simulink model "FlightSim"  (Simulink 7.9)
settings: Solver=ode45  StartTime=0.0  StopTime=10.0  RelTol=1e-3
undefined symbols (not defined in the file or in its folder): datcom_out, deg, ft, m, Newton, nfs, rad, Raphson, s, sigbuilder_block
libraries: aerolibconvert2 x12, aerolibadyn x2, aerolibasang x2, aerolibutil x1, simulink x1
(part 2 of 2)

== system FlightSim/6DoF Nonlinear Flight Equations of Motion (Rigid Body)/AngularAcceleration(Omegadot)/Cross Product/Subsystem3 ==
  A : Inport
  B : Inport  Port=2
  Demux : Demux  Outputs=3
  Demux1 : Demux  Outputs=3
  Mux : Mux  Inputs=3
  i x k : Product  SaturateOnIntegerOverflow=on  InputSameDT=on  OutDataTypeStr=Inherit: Same as first input
  j x i : Product  SaturateOnIntegerOverflow=on  InputSameDT=on  OutDataTypeStr=Inherit: Same as first input
  k x j : Product  SaturateOnIntegerOverflow=on  InputSameDT=on  OutDataTypeStr=Inherit: Same as first input
  Out2 : Outport
  wires:
  j x i/1 -> Mux/3
  i x k/1 -> Mux/2
  k x j/1 -> Mux/1
  Mux/1 -> Out2/1
  Demux1/1 -> j x i/2
  Demux/2 -> j x i/1
  Demux1/3 -> i x k/2
  Demux/1 -> i x k/1
  Demux1/2 -> k x j/2
  Demux/3 -> k x j/1
  B/1 -> Demux1/1
  A/1 -> Demux/1

== system FlightSim/6DoF Nonlinear Flight Equations of Motion (Rigid Body)/Linear Acceleration(Vdot)/Cross Product/Subsystem2 ==
  A : Inport
  B : Inport  Port=2
  Demux : Demux  Outputs=3
  Demux1 : Demux  Outputs=3
  Mux : Mux  Inputs=3
  i x j : Product  SaturateOnIntegerOverflow=on  InputSameDT=on  OutDataTypeStr=Inherit: Same as first input
  j x k : Product  SaturateOnIntegerOverflow=on  InputSameDT=on  OutDataTypeStr=Inherit: Same as first input
  k x i : Product  SaturateOnIntegerOverflow=on  InputSameDT=on  OutDataTypeStr=Inherit: Same as first input
  Out1 : Outport
  wires:
  Demux1/3 -> j x k/2
  Demux/2 -> j x k/1
  Demux/3 -> k x i/1
  Demux1/1 -> k x i/2
  Demux1/2 -> i x j/2
  Demux/1 -> i x j/1
  i x j/1 -> Mux/3
  k x i/1 -> Mux/2
  j x k/1 -> Mux/1
  B/1 -> Demux1/1
  A/1 -> Demux/1
  Mux/1 -> Out1/1

== system FlightSim/6DoF Nonlinear Flight Equations of Motion (Rigid Body)/Linear Acceleration(Vdot)/Cross Product/Subsystem3 ==
  A : Inport
  B : Inport  Port=2
  Demux : Demux  Outputs=3
  Demux1 : Demux  Outputs=3
  Mux : Mux  Inputs=3
  i x k : Product  SaturateOnIntegerOverflow=on  InputSameDT=on  OutDataTypeStr=Inherit: Same as first input
  j x i : Product  SaturateOnIntegerOverflow=on  InputSameDT=on  OutDataTypeStr=Inherit: Same as first input
  k x j : Product  SaturateOnIntegerOverflow=on  InputSameDT=on  OutDataTypeStr=Inherit: Same as first input
  Out2 : Outport
  wires:
  j x i/1 -> Mux/3
  i x k/1 -> Mux/2
  k x j/1 -> Mux/1
  Mux/1 -> Out2/1
  Demux1/1 -> j x i/2
  Demux/2 -> j x i/1
  Demux1/3 -> i x k/2
  Demux/1 -> i x k/1
  Demux1/2 -> k x j/2
  Demux/3 -> k x j/1
  B/1 -> Demux1/1
  A/1 -> Demux/1

== system FlightSim/Forces & Moments/Aerodynamic Forces and Moments/Aero Attributes/Dynamic Pressure Calc ==
  Air Density : Inport  PortDimensions=1
  Linear Velocity (Body) : Inport  Port=2  PortDimensions=[3 1]
  0.5*rh : Product  SaturateOnIntegerOverflow=on  InputSameDT=on  OutDataTypeStr=Inherit: Same as first input
  Dot Product : DotProduct  InputSameDT=on  OutDataTypeStr=Inherit: Inherit via internal rule
  Gain : Gain  Gain=0.5  SaturateOnIntegerOverflow=on  OutDataTypeStr=Inherit: Same as input  ParamDataTypeStr=Inherit: Same as input
  V^2 : Abs
  Dynamic Pressure : Outport
  wires:
  Dot Product/1 -> V^2/1
  Linear Velocity (Body)/1 -> Dot Product/2, Dot Product/1
  Air Density/1 -> Gain/1
  V^2/1 -> 0.5*rh/1
  Gain/1 -> 0.5*rh/2
  0.5*rh/1 -> Dynamic Pressure/1

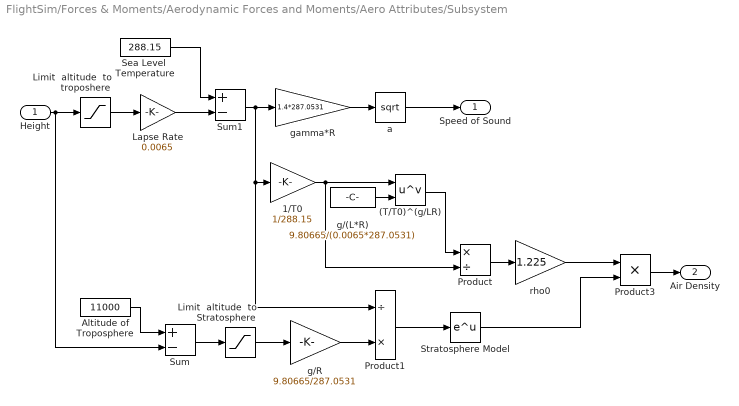
== system FlightSim/Forces & Moments/Aerodynamic Forces and Moments/Aero Attributes/Subsystem ==
  Height : Inport
  "(T/T0)^(g/LR) " : Math  Operator=pow  SaturateOnIntegerOverflow=on
  1/T0 : Gain  Gain=1/288.15  SaturateOnIntegerOverflow=on  OutDataTypeStr=Inherit: Same as input  ParamDataTypeStr=Inherit: Same as input
  Altitude of Troposphere : Constant  Value=11000  OutDataTypeStr=Inherit: Inherit via back propagation
  Lapse Rate : Gain  Gain=0.0065  SaturateOnIntegerOverflow=on  OutDataTypeStr=Inherit: Same as input  ParamDataTypeStr=Inherit: Same as input
  Limit  altitude  to Stratosphere : Saturate  UpperLimit=0  LowerLimit=11000-20000
  Limit  altitude  to troposhere : Saturate  UpperLimit=11000  LowerLimit=0
  Product : Product  Inputs=*/  SaturateOnIntegerOverflow=on  InputSameDT=on  OutDataTypeStr=Inherit: Same as first input
  Product1 : Product  Inputs=/*  SaturateOnIntegerOverflow=on  InputSameDT=on  OutDataTypeStr=Inherit: Same as first input
  Product3 : Product  SaturateOnIntegerOverflow=on  InputSameDT=on  OutDataTypeStr=Inherit: Same as first input
  Sea Level  Temperature : Constant  Value=288.15  OutDataTypeStr=Inherit: Inherit via back propagation
  Stratosphere Model : Math  SaturateOnIntegerOverflow=on
  Sum : Sum  Inputs=+-  SaturateOnIntegerOverflow=on  InputSameDT=on  OutDataTypeStr=Inherit: Same as first input
  Sum1 : Sum  Inputs=+-  SaturateOnIntegerOverflow=on  InputSameDT=on  OutDataTypeStr=Inherit: Same as first input
  a : Sqrt  AlgorithmType=Newton-Raphson  SaturateOnIntegerOverflow=on
  g/(L*R) : Constant  Value=9.80665/(0.0065*287.0531)  OutDataTypeStr=Inherit: Inherit via back propagation
  g/R : Gain  Gain=9.80665/287.0531  SaturateOnIntegerOverflow=on  OutDataTypeStr=Inherit: Same as input  ParamDataTypeStr=Inherit: Same as input
  gamma*R : Gain  Gain=1.4*287.0531  SaturateOnIntegerOverflow=on  OutDataTypeStr=Inherit: Same as input  ParamDataTypeStr=Inherit: Same as input
  rho0 : Gain  Gain=1.225  SaturateOnIntegerOverflow=on  OutDataTypeStr=Inherit: Same as input  ParamDataTypeStr=Inherit: Same as input
  Speed of Sound : Outport  PortDimensions=1
  Air Density : Outport  Port=2  PortDimensions=1
  wires:
  g/(L*R)/1 -> "(T/T0)^(g/LR) "/2
  Height/1 -> Limit  altitude  to troposhere/1, Sum/2
  Limit  altitude  to troposhere/1 -> Lapse Rate/1
  Product/1 -> rho0/1
  "(T/T0)^(g/LR) "/1 -> Product/1
  1/T0/1 -> "(T/T0)^(g/LR) "/1, Product/2
  gamma*R/1 -> a/1
  a/1 -> Speed of Sound/1
  Sum1/1 -> gamma*R/1, 1/T0/1, Product1/1
  Lapse Rate/1 -> Sum1/2
  Sea Level  Temperature/1 -> Sum1/1
  rho0/1 -> Product3/1
  Product3/1 -> Air Density/1
  Stratosphere Model/1 -> Product3/2
  g/R/1 -> Product1/2
  Product1/1 -> Stratosphere Model/1
  Altitude of Troposphere/1 -> Sum/1
  Sum/1 -> Limit  altitude  to Stratosphere/1
  Limit  altitude  to Stratosphere/1 -> g/R/1

== system FlightSim/Forces & Moments/Aerodynamic Forces and Moments/Aero Attributes/Velocity Magnitude ==
  Velocity : Inport
  Dot Product : DotProduct  InputSameDT=on  OutDataTypeStr=Inherit: Inherit via internal rule
  Sqrt : Sqrt  SaturateOnIntegerOverflow=on
  Velocity Magnitude : Outport
  wires:
  Sqrt/1 -> Velocity Magnitude/1  "abs(V)"
  Velocity/1 -> Dot Product/2, Dot Product/1
  Dot Product/1 -> Sqrt/1

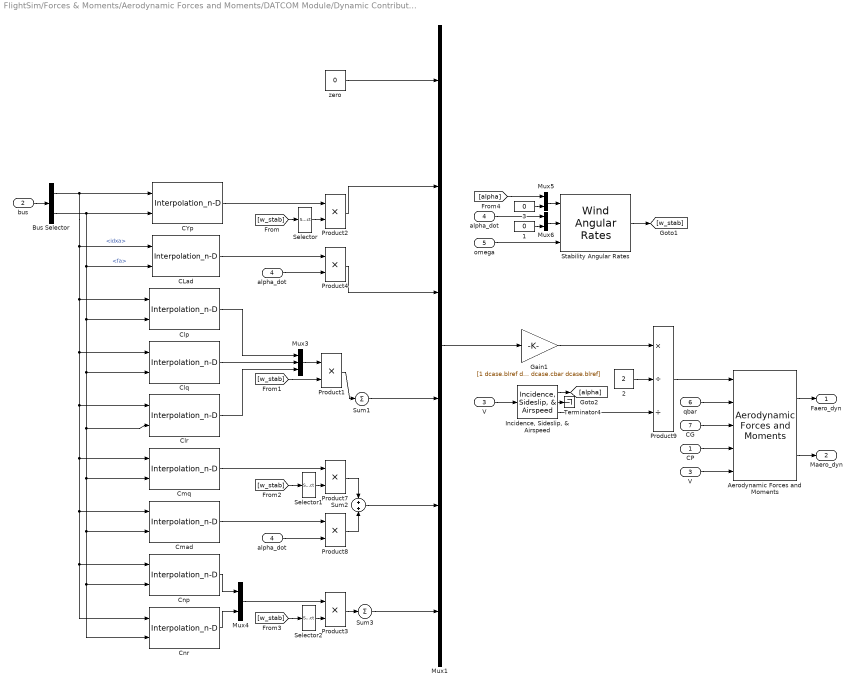
== system FlightSim/Forces & Moments/Aerodynamic Forces and Moments/DATCOM Module/Dynamic Contribution ==
  CP : Inport
  bus : Inport  Port=2
  V : Inport  Port=3
  alpha_dot : Inport  Port=4
  omega : Inport  Port=5
  qbar : Inport  Port=6
  CG : Inport  Port=7
  " V " : InportShadow  Port=3
  " alpha_dot " : InportShadow  Port=4
  1 : Constant  Value=0
  2 : Constant  Value=2
  3 : Constant  Value=0
  Aerodynamic Forces and Moments : aerolibadyn/Aerodynamic Forces and Moments   inputAxes=Stability  outputForceAxes=Body  outputMomentAxes=Body  S=dcase.sref  b=dcase.blref  cbar=dcase.cbar
  Bus Selector : BusSelector  OutputSignals=idxa,fa
  CLad : Interpolation_n-D  NumberOfTableDimensions=1  Table="permute(dcase.clad,[1  2])"  OutDataTypeStr=double
      settings: InputPortMap=u0,u1
  CYp : Interpolation_n-D  NumberOfTableDimensions=1  Table="permute(dcase.cyp,[1  2])"  OutDataTypeStr=double
      settings: InputPortMap=u0,u1
  Clp : Interpolation_n-D  NumberOfTableDimensions=1  Table="permute(dcase.clp,[1  2])"  OutDataTypeStr=double
      settings: InputPortMap=u0,u1
  Clq : Interpolation_n-D  NumberOfTableDimensions=1  Table="permute(dcase.clq,[1  2])"  OutDataTypeStr=double
      settings: InputPortMap=u0,u1
  Clr : Interpolation_n-D  NumberOfTableDimensions=1  Table="permute(dcase.clr,[1  2])"  OutDataTypeStr=double
      settings: InputPortMap=u0,u1
  Cmad : Interpolation_n-D  NumberOfTableDimensions=1  Table="permute(dcase.cmad,[1  2])"  OutDataTypeStr=double
      settings: InputPortMap=u0,u1
  Cmq : Interpolation_n-D  NumberOfTableDimensions=1  Table="permute(dcase.cmq,[1  2])"  OutDataTypeStr=double
      settings: InputPortMap=u0,u1
  Cnp : Interpolation_n-D  NumberOfTableDimensions=1  Table="permute(dcase.cnp,[1  2])"  OutDataTypeStr=double
      settings: InputPortMap=u0,u1
  Cnr : Interpolation_n-D  NumberOfTableDimensions=1  Table="permute(dcase.cnr,[1  2])"  OutDataTypeStr=double
      settings: InputPortMap=u0,u1
  Gain1 : Gain  Gain=[1 dcase.blref dcase.cbar dcase.blref dcase.cbar dcase.blref]
  "Incidence, Sideslip, & Airspeed" : aerolibasang/Incidence, Sideslip, & Airspeed
  Mux1 : Mux  Inputs=6
  Mux3 : Mux  Inputs=3
  Mux4 : Mux  Inputs=2
  Mux5 : Mux  Inputs=2
  Mux6 : Mux  Inputs=2
  Product{1..4,7..8} (6 alike) : Product  RndMeth=Zero
  Product9 : Product  Inputs=*//  RndMeth=Zero
  Selector : Selector  InputPortWidth=3  IndexOptions=Index vector (dialog)  Indices=1  OutputSizes=1
  Selector1 : Selector  InputPortWidth=3  IndexOptions=Index vector (dialog)  Indices=2  OutputSizes=1
  Selector2 : Selector  InputPortWidth=3  IndexOptions=Index vector (dialog)  Indices=[1 3]  OutputSizes=1
  Stability Angular Rates : aerolibasang/Wind Angular Rates
  Sum1 : Sum  Inputs=+
  Sum2 : Sum  Inputs=+|+
  Sum3 : Sum  Inputs=+
  Terminator4 : Terminator
  "alpha_dot " : InportShadow  Port=4
  zero : Constant  Value=0
  Faero_dyn : Outport
  Maero_dyn : Outport  Port=2
  wires:
  bus/1 -> Bus Selector/1
  Mux1/1 -> Gain1/1
  CLad/1 -> Product4/1
  Cnp/1 -> Mux4/1
  Cmq/1 -> Product7/1
  Sum1/1 -> Mux1/4
  Clq/1 -> Mux3/2
  Selector/1 -> Product2/2
  CYp/1 -> Product2/1
  "alpha_dot "/1 -> Product4/2
  [w_stab] -> Selector/1
  Clr/1 -> Mux3/3
  Clp/1 -> Mux3/1
  Mux3/1 -> Product1/1
  [w_stab] -> Product1/2
  Product1/1 -> Sum1/1
  [w_stab] -> Selector1/1
  Selector1/1 -> Product7/2
  Product7/1 -> Sum2/1
  Cmad/1 -> Product8/1
  Product8/1 -> Sum2/2
  alpha_dot/1 -> Product8/2
  Cnr/1 -> Mux4/2
  [w_stab] -> Selector2/1
  Mux4/1 -> Product3/1
  Selector2/1 -> Product3/2
  Sum3/1 -> Mux1/6
  Product3/1 -> Sum3/1
  Gain1/1 -> Product9/1
  Product9/1 -> Aerodynamic Forces and Moments/1
  2/1 -> Product9/2
  V/1 -> "Incidence, Sideslip, & Airspeed"/1
  omega/1 -> Stability Angular Rates/3
  Sum2/1 -> Mux1/5
  Product4/1 -> Mux1/3
  zero/1 -> Mux1/1
  "Incidence, Sideslip, & Airspeed"/3 -> Product9/3
  "Incidence, Sideslip, & Airspeed"/2 -> Terminator4/1
  "Incidence, Sideslip, & Airspeed"/1 -> [alpha]
  Aerodynamic Forces and Moments/1 -> Faero_dyn/1
  qbar/1 -> Aerodynamic Forces and Moments/2
  Aerodynamic Forces and Moments/2 -> Maero_dyn/1
  " V "/1 -> Aerodynamic Forces and Moments/5
  Stability Angular Rates/1 -> [w_stab]
  [alpha] -> Mux5/1
  Mux5/1 -> Stability Angular Rates/1
  Mux6/1 -> Stability Angular Rates/2
  " alpha_dot "/1 -> Mux6/1
  1/1 -> Mux6/2
  CG/1 -> Aerodynamic Forces and Moments/3
  CP/1 -> Aerodynamic Forces and Moments/4
  Bus Selector/1 -> CYp/1, CLad/1, Cnr/1, Cnp/1, Cmad/1, Cmq/1, Clr/1, Clq/1, Clp/1  "<idxa>"
  Bus Selector/2 -> CYp/2, CLad/2, Cnr/2, Cnp/2, Cmad/2, Cmq/2, Clr/2, Clq/2, Clp/2  "<fa>"
  3/1 -> Mux5/2
  Product2/1 -> Mux1/2

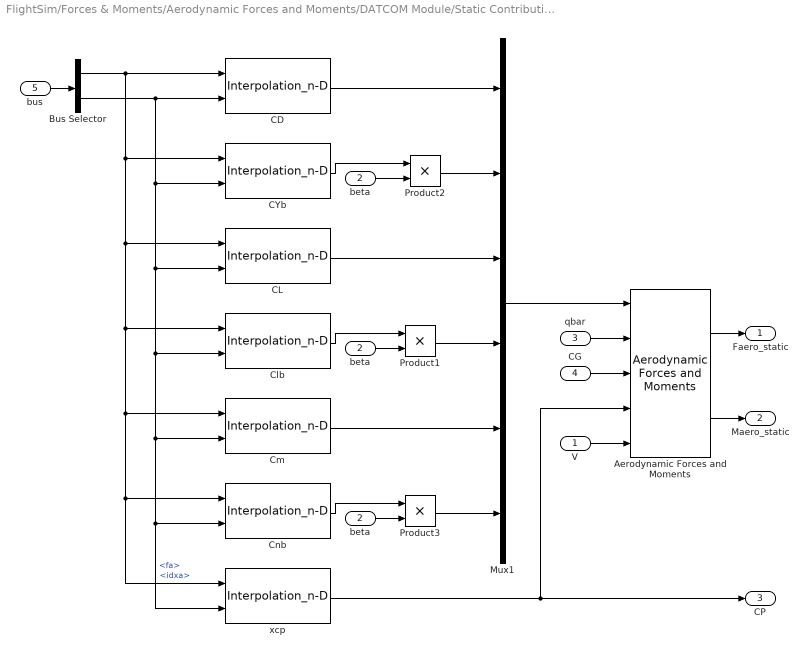
== system FlightSim/Forces & Moments/Aerodynamic Forces and Moments/DATCOM Module/Static Contribution ==
  "V " : Inport
  beta : Inport  Port=2
  qbar : Inport  Port=3
  CG : Inport  Port=4
  bus : Inport  Port=5
  " beta " : InportShadow  Port=2
  Aerodynamic Forces and Moments : aerolibadyn/Aerodynamic Forces and Moments   inputAxes=Stability  outputForceAxes=Body  outputMomentAxes=Body  S=dcase.sref  b=dcase.blref  cbar=dcase.cbar
  Bus Selector : BusSelector  OutputSignals=idxa,fa
  CD : Interpolation_n-D  NumberOfTableDimensions=1  Table=dcase.cd  OutDataTypeStr=double
      settings: InputPortMap=u0,u1
  CL : Interpolation_n-D  NumberOfTableDimensions=1  Table=dcase.cl  OutDataTypeStr=double
      settings: InputPortMap=u0,u1
  CYb : Interpolation_n-D  NumberOfTableDimensions=1  Table=dcase.cyb  OutDataTypeStr=double
      settings: InputPortMap=u0,u1
  Clb : Interpolation_n-D  NumberOfTableDimensions=1  Table=dcase.clb  OutDataTypeStr=double
      settings: InputPortMap=u0,u1
  Cm : Interpolation_n-D  NumberOfTableDimensions=1  Table=dcase.cm  OutDataTypeStr=double
      settings: InputPortMap=u0,u1
  Cnb : Interpolation_n-D  NumberOfTableDimensions=1  Table=dcase.cnb  OutDataTypeStr=double
      settings: InputPortMap=u0,u1
  Mux1 : Mux  Inputs=6
  Product1 : Product  RndMeth=Zero
  Product2 : Product  RndMeth=Zero
  Product3 : Product  RndMeth=Zero
  "beta " : InportShadow  Port=2
  xcp : Interpolation_n-D  NumberOfTableDimensions=1  Table=dcase.xcp  OutDataTypeStr=double
      settings: InputPortMap=u0,u1
  Faero_static : Outport
  Maero_static : Outport  Port=2
  "CP " : Outport  Port=3
  wires:
  CG/1 -> Aerodynamic Forces and Moments/3
  bus/1 -> Bus Selector/1
  Bus Selector/1 -> CD/1, CYb/1, Clb/1, Cm/1, Cnb/1, xcp/1, CL/1  "<idxa>"
  Bus Selector/2 -> CD/2, CYb/2, Clb/2, Cm/2, Cnb/2, xcp/2, CL/2  "<fa>"
  CD/1 -> Mux1/1
  CL/1 -> Mux1/3
  CYb/1 -> Product2/1
  beta/1 -> Product2/2
  Clb/1 -> Product1/1
  "beta "/1 -> Product1/2
  Product2/1 -> Mux1/2
  Product1/1 -> Mux1/4
  Cm/1 -> Mux1/5
  Cnb/1 -> Product3/1
  " beta "/1 -> Product3/2
  Product3/1 -> Mux1/6
  Mux1/1 -> Aerodynamic Forces and Moments/1
  Aerodynamic Forces and Moments/1 -> Faero_static/1
  qbar/1 -> Aerodynamic Forces and Moments/2
  Aerodynamic Forces and Moments/2 -> Maero_static/1
  "V "/1 -> Aerodynamic Forces and Moments/5
  xcp/1 -> "CP "/1, Aerodynamic Forces and Moments/4

== system FlightSim/Forces & Moments/Moments/Pitch Moment Coefficient/Velocity Magnitude ==
  Velocity : Inport
  Dot Product : DotProduct  InputSameDT=on  OutDataTypeStr=Inherit: Inherit via internal rule
  Sqrt : Sqrt  SaturateOnIntegerOverflow=on
  Velocity Magnitude : Outport
  wires:
  Sqrt/1 -> Velocity Magnitude/1  "abs(V)"
  Velocity/1 -> Dot Product/2, Dot Product/1
  Dot Product/1 -> Sqrt/1

== system FlightSim/Forces & Moments/Moments/Roll Moment Coefficient/Velocity Magnitude ==
  Velocity : Inport
  Dot Product : DotProduct  InputSameDT=on  OutDataTypeStr=Inherit: Inherit via internal rule
  Sqrt : Sqrt  SaturateOnIntegerOverflow=on
  Velocity Magnitude : Outport
  wires:
  Sqrt/1 -> Velocity Magnitude/1  "abs(V)"
  Velocity/1 -> Dot Product/2, Dot Product/1
  Dot Product/1 -> Sqrt/1

== system FlightSim/Forces & Moments/Moments/Yaw Moment Coefficient/Velocity Magnitude ==
  Velocity : Inport
  Dot Product : DotProduct  InputSameDT=on  OutDataTypeStr=Inherit: Inherit via internal rule
  Sqrt : Sqrt  SaturateOnIntegerOverflow=on
  Velocity Magnitude : Outport
  wires:
  Sqrt/1 -> Velocity Magnitude/1  "abs(V)"
  Velocity/1 -> Dot Product/2, Dot Product/1
  Dot Product/1 -> Sqrt/1

== system FlightSim/Forces & Moments/Repository/Control Forces/Aerodynamic  Force ==
  CL : Inport  PortDimensions=1
  CD : Inport  Port=2  PortDimensions=1
  CY : Inport  Port=3  PortDimensions=1
  Dynamic Pressure : Inport  Port=4  PortDimensions=1
  Alpha : Inport  Port=5  PortDimensions=1
  Beta : Inport  Port=6  PortDimensions=1
  ChSign : Gain  Gain=-1  SaturateOnIntegerOverflow=on  OutDataTypeStr=Inherit: Same as input  ParamDataTypeStr=Inherit: Same as input
  ChSign1 : Gain  Gain=-1  SaturateOnIntegerOverflow=on  OutDataTypeStr=Inherit: Same as input  ParamDataTypeStr=Inherit: Same as input
  Mux : Mux  Inputs=3
  Product{,2..4} (4 alike) : Product  SaturateOnIntegerOverflow=on  InputSameDT=on  OutDataTypeStr=Inherit: Same as first input
  Product1 : Product  Multiplication=Matrix(*)  SaturateOnIntegerOverflow=on  InputSameDT=on  OutDataTypeStr=Inherit: Same as first input
  Wind2Body TM : Subsystem
  Wing Area : Constant  Value=wing_area
  Aerodynamic Force : Outport  PortDimensions=[3,1]
  wires:
  Wind2Body TM/1(T_BW) -> Product1/1
  Product1/1 -> Aerodynamic Force/1
  Beta/1 -> Wind2Body TM/2(Beta)
  CD/1 -> ChSign/1
  CL/1 -> ChSign1/1
  Alpha/1 -> Wind2Body TM/1(Alpha)
  Dynamic Pressure/1 -> Product/1
  Wing Area/1 -> Product/2
  Product/1 -> Product2/1, Product3/1, Product4/1
  ChSign/1 -> Product2/2
  CY/1 -> Product3/2
  ChSign1/1 -> Product4/2
  Product2/1 -> Mux/1
  Product3/1 -> Mux/2
  Product4/1 -> Mux/3
  Mux/1 -> Product1/2

== system FlightSim/Forces & Moments/Repository/Control Forces/Drag Coefficient ==
  DeltaElevator : Inport  PortDimensions=1
  DeltaFlap : Inport  Port=2  PortDimensions=1
  DeltaAileron : Inport  Port=3  PortDimensions=1
  DeltaRudder : Inport  Port=4  PortDimensions=1
  Abs{,1..3} (4 alike) : Abs  SaturateOnIntegerOverflow=on
  Sum2 : Sum  Inputs=++++  SaturateOnIntegerOverflow=on  InputSameDT=on  OutDataTypeStr=Inherit: Same as first input
  cDdelta_a : Lookup_n-D  NumberOfTableDimensions=1  BreakpointsForDimension1=cDdelta_a(:,1)  Table=cDdelta_a(:,2)  RndMeth=Simplest  InputSameDT=on
  cDdelta_e : Lookup_n-D  NumberOfTableDimensions=1  BreakpointsForDimension1=cDdelta_e(:,1)  Table=cDdelta_e(:,2)  RndMeth=Simplest  InputSameDT=on
  cDdelta_f : Lookup_n-D  NumberOfTableDimensions=1  BreakpointsForDimension1=cDdelta_f(:,1)  Table=cDdelta_f(:,2)  RndMeth=Simplest  InputSameDT=on
  cDdelta_f3 : Lookup_n-D  NumberOfTableDimensions=1  BreakpointsForDimension1=cDdelta_r(:,1)  Table=cDdelta_r(:,2)  RndMeth=Simplest  InputSameDT=on
  CD : Outport  PortDimensions=1
  wires:
  Sum2/1 -> CD/1
  DeltaRudder/1 -> cDdelta_f3/1
  DeltaAileron/1 -> cDdelta_a/1
  DeltaElevator/1 -> cDdelta_e/1
  DeltaFlap/1 -> cDdelta_f/1
  cDdelta_f3/1 -> Abs3/1
  cDdelta_a/1 -> Abs2/1
  cDdelta_e/1 -> Abs1/1
  cDdelta_f/1 -> Abs/1
  Abs2/1 -> Sum2/3
  Abs3/1 -> Sum2/4
  Abs1/1 -> Sum2/1
  Abs/1 -> Sum2/2

== system FlightSim/Forces & Moments/Repository/Control Forces/Lift Coefficient ==
  DeltaElevator : Inport  PortDimensions=1
  DeltaFlap : Inport  Port=2  PortDimensions=1
  Sum3 : Sum  SaturateOnIntegerOverflow=on  InputSameDT=on  OutDataTypeStr=Inherit: Same as first input
  cLdelta_e : Lookup_n-D  NumberOfTableDimensions=1  BreakpointsForDimension1=cLdelta_e(:,1)  Table=cLdelta_e(:,2)  RndMeth=Simplest  InputSameDT=on
  cLdelta_f : Lookup_n-D  NumberOfTableDimensions=1  BreakpointsForDimension1=cLdelta_f(:,1)  Table=cLdelta_f(:,2)  RndMeth=Simplest  InputSameDT=on
  CL : Outport  PortDimensions=1
  wires:
  Sum3/1 -> CL/1
  cLdelta_f/1 -> Sum3/2
  cLdelta_e/1 -> Sum3/1
  DeltaFlap/1 -> cLdelta_f/1
  DeltaElevator/1 -> cLdelta_e/1

== system FlightSim/Forces & Moments/Repository/Control Forces/SideForce Coefficient ==
  DeltaAileron : Inport  PortDimensions=1
  DeltaRudder : Inport  Port=2  PortDimensions=1
  Sum2 : Sum  SaturateOnIntegerOverflow=on  InputSameDT=on  OutDataTypeStr=Inherit: Same as first input
  cYdelta_a : Lookup_n-D  NumberOfTableDimensions=1  BreakpointsForDimension1=cYdelta_a(:,1)  Table=cYdelta_a(:,2)  RndMeth=Simplest  InputSameDT=on
  cYdelta_r : Lookup_n-D  NumberOfTableDimensions=1  BreakpointsForDimension1=cYdelta_r(:,1)  Table=cYdelta_r(:,2)  RndMeth=Simplest  InputSameDT=on
  CY : Outport
  wires:
  Sum2/1 -> CY/1
  DeltaRudder/1 -> cYdelta_r/1
  DeltaAileron/1 -> cYdelta_a/1
  cYdelta_a/1 -> Sum2/1
  cYdelta_r/1 -> Sum2/2

== system FlightSim/Forces & Moments/Repository/Control Moments/Aerodynamic Moment  ==
  Cl : Inport
  Cm : Inport  Port=2
  Cn : Inport  Port=3
  Dynamic Pressure : Inport  Port=4
  Dynamic Pressure1 : InportShadow  Port=4
  Dynamic Pressure2 : InportShadow  Port=4
  Mux : Mux  Inputs=3
  Pitch : Product  Inputs=4  SaturateOnIntegerOverflow=on  InputSameDT=on  OutDataTypeStr=Inherit: Same as first input
  Roll : Product  Inputs=4  SaturateOnIntegerOverflow=on  InputSameDT=on  OutDataTypeStr=Inherit: Same as first input
  Wing area : Constant  Value=refarea
  Wing chord : Constant  Value=meanchord
  Wing span : Constant  Value=span
  Wing span2 : Constant  Value=span
  Yaw : Product  Inputs=4  SaturateOnIntegerOverflow=on  InputSameDT=on  OutDataTypeStr=Inherit: Same as first input
  Aerodynamic Moment : Outport  PortDimensions=[3,1]
  wires:
  Wing span/1 -> Roll/3
  Wing chord/1 -> Pitch/3
  Dynamic Pressure/1 -> Roll/1
  Cn/1 -> Yaw/4
  Cm/1 -> Pitch/4
  Cl/1 -> Roll/4
  Dynamic Pressure1/1 -> Pitch/1
  Dynamic Pressure2/1 -> Yaw/1
  Wing span2/1 -> Yaw/3
  Wing area/1 -> Pitch/2, Roll/2, Yaw/2
  Mux/1 -> Aerodynamic Moment/1
  Roll/1 -> Mux/1
  Pitch/1 -> Mux/2
  Yaw/1 -> Mux/3

== system FlightSim/Forces & Moments/Repository/Control Moments/Pitch Moment Coefficient ==
  DeltaElevator : Inport
  DeltaFlap : Inport  Port=2
  Sum2 : Sum  SaturateOnIntegerOverflow=on  InputSameDT=on  OutDataTypeStr=Inherit: Same as first input
  cmdelta_e : Lookup_n-D  NumberOfTableDimensions=1  BreakpointsForDimension1=cmdelta_e(:,1)  Table=cmdelta_e(:,2)  RndMeth=Simplest  InputSameDT=on
  cmdelta_f : Lookup_n-D  NumberOfTableDimensions=1  BreakpointsForDimension1=cmdelta_f(:,1)  Table=cmdelta_f(:,2)  RndMeth=Simplest  InputSameDT=on
  Cm : Outport  PortDimensions=1
  wires:
  DeltaFlap/1 -> cmdelta_f/1
  DeltaElevator/1 -> cmdelta_e/1
  Sum2/1 -> Cm/1
  cmdelta_f/1 -> Sum2/1
  cmdelta_e/1 -> Sum2/2

== system FlightSim/Forces & Moments/Repository/Control Moments/Roll Moment Coefficient ==
  DeltaAileron : Inport
  DeltaRudder : Inport  Port=2
  Sum2 : Sum  SaturateOnIntegerOverflow=on  InputSameDT=on  OutDataTypeStr=Inherit: Same as first input
  cldelta_a : Lookup_n-D  NumberOfTableDimensions=1  BreakpointsForDimension1=cldelta_a(:,1)  Table=cldelta_a(:,2)  RndMeth=Simplest  InputSameDT=on
  cldelta_r : Lookup_n-D  NumberOfTableDimensions=1  BreakpointsForDimension1=cldelta_r(:,1)  Table=cldelta_r(:,2)  RndMeth=Simplest  InputSameDT=on
  Cl : Outport  PortDimensions=1
  wires:
  DeltaAileron/1 -> cldelta_a/1
  DeltaRudder/1 -> cldelta_r/1
  Sum2/1 -> Cl/1
  cldelta_a/1 -> Sum2/1
  cldelta_r/1 -> Sum2/2

== system FlightSim/Forces & Moments/Repository/Control Moments/Yaw Moment Coefficient ==
  DeltaAileron : Inport
  DeltaRudder : Inport  Port=2
  Sum2 : Sum  SaturateOnIntegerOverflow=on  InputSameDT=on  OutDataTypeStr=Inherit: Same as first input
  cndelta_a1 : Lookup_n-D  NumberOfTableDimensions=1  BreakpointsForDimension1=cndelta_a(:,1)  Table=cndelta_a(:,2)  RndMeth=Simplest  InputSameDT=on
  cndelta_r2 : Lookup_n-D  NumberOfTableDimensions=1  BreakpointsForDimension1=cndelta_r(:,1)  Table=cndelta_r(:,2)  RndMeth=Simplest  InputSameDT=on
  Cn : Outport  PortDimensions=1
  wires:
  DeltaAileron/1 -> cndelta_a1/1
  DeltaRudder/1 -> cndelta_r2/1
  Sum2/1 -> Cn/1
  cndelta_a1/1 -> Sum2/1
  cndelta_r2/1 -> Sum2/2

== system FlightSim/Forces & Moments/Repository/Forces/Aerodynamic  Force ==
  CL : Inport  PortDimensions=1
  CD : Inport  Port=2  PortDimensions=1
  CY : Inport  Port=3  PortDimensions=1
  Dynamic Pressure : Inport  Port=4  PortDimensions=1
  Alpha : Inport  Port=5  PortDimensions=1
  Beta : Inport  Port=6  PortDimensions=1
  ChSign : Gain  Gain=-1  SaturateOnIntegerOverflow=on  OutDataTypeStr=Inherit: Same as input  ParamDataTypeStr=Inherit: Same as input
  ChSign1 : Gain  Gain=-1  SaturateOnIntegerOverflow=on  OutDataTypeStr=Inherit: Same as input  ParamDataTypeStr=Inherit: Same as input
  Mux : Mux  Inputs=3
  Product{,2..4} (4 alike) : Product  SaturateOnIntegerOverflow=on  InputSameDT=on  OutDataTypeStr=Inherit: Same as first input
  Product1 : Product  Multiplication=Matrix(*)  SaturateOnIntegerOverflow=on  InputSameDT=on  OutDataTypeStr=Inherit: Same as first input
  Wind2Body TM : Subsystem
  Wing Area : Constant  Value=nfs.refarea
  Aerodynamic Force : Outport  PortDimensions=[3,1]
  wires:
  Wind2Body TM/1(T_BW) -> Product1/1
  Product1/1 -> Aerodynamic Force/1
  Beta/1 -> Wind2Body TM/2(Beta)
  CD/1 -> ChSign/1
  CL/1 -> ChSign1/1
  Alpha/1 -> Wind2Body TM/1(Alpha)
  Dynamic Pressure/1 -> Product/1
  Wing Area/1 -> Product/2
  Product/1 -> Product2/1, Product3/1, Product4/1
  ChSign/1 -> Product2/2
  CY/1 -> Product3/2
  ChSign1/1 -> Product4/2
  Product2/1 -> Mux/1
  Product3/1 -> Mux/2
  Product4/1 -> Mux/3
  Mux/1 -> Product1/2

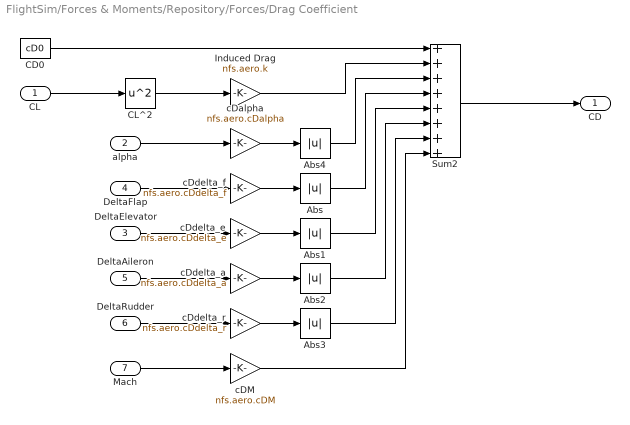
== system FlightSim/Forces & Moments/Repository/Forces/Drag Coefficient ==
  CL : Inport  PortDimensions=1
  alpha : Inport  Port=2  PortDimensions=1
  DeltaElevator : Inport  Port=3  PortDimensions=1
  DeltaFlap : Inport  Port=4  PortDimensions=1
  DeltaAileron : Inport  Port=5  PortDimensions=1
  DeltaRudder : Inport  Port=6  PortDimensions=1
  Mach : Inport  Port=7  PortDimensions=1
  Abs{,1..4} (5 alike) : Abs  SaturateOnIntegerOverflow=on
  CD0 : Constant  Value=cD0
  CL^2 : Math  Operator=square  SaturateOnIntegerOverflow=on
  Induced Drag : Gain  Gain=nfs.aero.k  SaturateOnIntegerOverflow=on  OutDataTypeStr=Inherit: Same as input  ParamDataTypeStr=Inherit: Same as input
  Sum2 : Sum  Inputs=++++++++  SaturateOnIntegerOverflow=on  InputSameDT=on  OutDataTypeStr=Inherit: Same as first input
  cDM : Gain  Gain=nfs.aero.cDM  SaturateOnIntegerOverflow=on  OutDataTypeStr=Inherit: Same as input  ParamDataTypeStr=Inherit: Same as input
  cDalpha : Gain  Gain=nfs.aero.cDalpha  SaturateOnIntegerOverflow=on  OutDataTypeStr=Inherit: Same as input  ParamDataTypeStr=Inherit: Same as input
  cDdelta_a : Gain  Gain=nfs.aero.cDdelta_a  SaturateOnIntegerOverflow=on  OutDataTypeStr=Inherit: Same as input  ParamDataTypeStr=Inherit: Same as input
  cDdelta_e : Gain  Gain=nfs.aero.cDdelta_e  SaturateOnIntegerOverflow=on  OutDataTypeStr=Inherit: Same as input  ParamDataTypeStr=Inherit: Same as input
  cDdelta_f : Gain  Gain=nfs.aero.cDdelta_f  SaturateOnIntegerOverflow=on  OutDataTypeStr=Inherit: Same as input  ParamDataTypeStr=Inherit: Same as input
  cDdelta_r : Gain  Gain=nfs.aero.cDdelta_r  SaturateOnIntegerOverflow=on  OutDataTypeStr=Inherit: Same as input  ParamDataTypeStr=Inherit: Same as input
  CD : Outport  PortDimensions=1
  wires:
  Sum2/1 -> CD/1
  DeltaRudder/1 -> cDdelta_r/1
  DeltaAileron/1 -> cDdelta_a/1
  DeltaElevator/1 -> cDdelta_e/1
  DeltaFlap/1 -> cDdelta_f/1
  Mach/1 -> cDM/1
  CL/1 -> CL^2/1
  cDdelta_r/1 -> Abs3/1
  cDdelta_a/1 -> Abs2/1
  cDdelta_e/1 -> Abs1/1
  cDdelta_f/1 -> Abs/1
  Induced Drag/1 -> Sum2/2
  CD0/1 -> Sum2/1
  CL^2/1 -> Induced Drag/1
  alpha/1 -> cDalpha/1
  cDalpha/1 -> Abs4/1
  Abs/1 -> Sum2/4
  Abs1/1 -> Sum2/5
  Abs2/1 -> Sum2/6
  Abs3/1 -> Sum2/7
  cDM/1 -> Sum2/8
  Abs4/1 -> Sum2/3

== system FlightSim/Forces & Moments/Repository/Forces/Lift Coefficient ==
  Linear Velocity : Inport  PortDimensions=[3 1]
  Alpha : Inport  Port=2  PortDimensions=1
  DeltaElevator : Inport  Port=3  PortDimensions=1
  DeltaFlap : Inport  Port=4  PortDimensions=1
  Alphadot : Inport  Port=5  PortDimensions=1
  Q : Inport  Port=6  PortDimensions=1
  Mach : Inport  Port=7  PortDimensions=1
  1 : Gain  Gain=2  SaturateOnIntegerOverflow=on  OutDataTypeStr=Inherit: Same as input  ParamDataTypeStr=Inherit: Same as input
  CL*c/(2V) : Product  Inputs=**/  SaturateOnIntegerOverflow=on  InputSameDT=on  OutDataTypeStr=Inherit: Same as first input
  CL0 : Constant  Value=cL0
  CLM : Gain  Gain=nfs.aero.cLM  SaturateOnIntegerOverflow=on  OutDataTypeStr=Inherit: Same as input  ParamDataTypeStr=Inherit: Same as input
  Sum1 : Sum  SaturateOnIntegerOverflow=on  InputSameDT=on  OutDataTypeStr=Inherit: Same as first input
  Sum3 : Sum  Inputs=++++++  SaturateOnIntegerOverflow=on  InputSameDT=on  OutDataTypeStr=Inherit: Same as first input
  Velocity Magnitude : Subsystem
  Wing chord1 : Constant  Value=meanchord
  cLalpha : Gain  Gain=nfs.aero.cLalpha  SaturateOnIntegerOverflow=on  OutDataTypeStr=Inherit: Same as input  ParamDataTypeStr=Inherit: Same as input
  cLalphadot : Gain  Gain=nfs.aero.cLalphadot  SaturateOnIntegerOverflow=on  OutDataTypeStr=Inherit: Same as input  ParamDataTypeStr=Inherit: Same as input
  cLdelta_e : Gain  Gain=nfs.aero.cLdelta_e  SaturateOnIntegerOverflow=on  OutDataTypeStr=Inherit: Same as input  ParamDataTypeStr=Inherit: Same as input
  cLdelta_f : Gain  Gain=nfs.aero.cLdelta_f  SaturateOnIntegerOverflow=on  OutDataTypeStr=Inherit: Same as input  ParamDataTypeStr=Inherit: Same as input
  cLq : Gain  Gain=nfs.aero.cLq  SaturateOnIntegerOverflow=on  OutDataTypeStr=Inherit: Same as input  ParamDataTypeStr=Inherit: Same as input
  CL : Outport  PortDimensions=1
  wires:
  Sum3/1 -> CL/1
  Q/1 -> cLq/1
  Alphadot/1 -> cLalphadot/1
  Velocity Magnitude/1(Velocity Magnitude) -> 1/1
  Linear Velocity/1 -> Velocity Magnitude/1(Velocity)
  Mach/1 -> CLM/1
  CL*c/(2V)/1 -> Sum3/5
  cLdelta_f/1 -> Sum3/4
  cLdelta_e/1 -> Sum3/3
  cLalpha/1 -> Sum3/2
  CL0/1 -> Sum3/1
  Sum1/1 -> CL*c/(2V)/1
  cLalphadot/1 -> Sum1/1
  DeltaFlap/1 -> cLdelta_f/1
  DeltaElevator/1 -> cLdelta_e/1
  Alpha/1 -> cLalpha/1
  cLq/1 -> Sum1/2
  Wing chord1/1 -> CL*c/(2V)/2
  1/1 -> CL*c/(2V)/3
  CLM/1 -> Sum3/6

== system FlightSim/Forces & Moments/Repository/Forces/SideForce Coefficient ==
  Linear Velocity : Inport  PortDimensions=[3 1]
  Beta : Inport  Port=2  PortDimensions=1
  P : Inport  Port=3  PortDimensions=1
  R : Inport  Port=4  PortDimensions=1
  DeltaAileron : Inport  Port=5  PortDimensions=1
  DeltaRudder : Inport  Port=6  PortDimensions=1
  2 : Gain  Gain=2  SaturateOnIntegerOverflow=on  OutDataTypeStr=Inherit: Same as input  ParamDataTypeStr=Inherit: Same as input
  CY*b/(2V) : Product  Inputs=**/  SaturateOnIntegerOverflow=on  InputSameDT=on  OutDataTypeStr=Inherit: Same as first input
  Sum : Sum  SaturateOnIntegerOverflow=on  InputSameDT=on  OutDataTypeStr=Inherit: Same as first input
  Sum2 : Sum  Inputs=++++  SaturateOnIntegerOverflow=on  InputSameDT=on  OutDataTypeStr=Inherit: Same as first input
  Velocity Magnitude : Subsystem
  Wing span : Constant  Value=nfs.span
  cYbeta : Gain  Gain=nfs.aero.cYbeta  SaturateOnIntegerOverflow=on  OutDataTypeStr=Inherit: Same as input  ParamDataTypeStr=Inherit: Same as input
  cYdelta_a : Gain  Gain=nfs.aero.cYdelta_a  SaturateOnIntegerOverflow=on  OutDataTypeStr=Inherit: Same as input  ParamDataTypeStr=Inherit: Same as input
  cYdelta_r : Gain  Gain=nfs.aero.cYdelta_r  SaturateOnIntegerOverflow=on  OutDataTypeStr=Inherit: Same as input  ParamDataTypeStr=Inherit: Same as input
  cYp : Gain  Gain=nfs.aero.cYp  SaturateOnIntegerOverflow=on  OutDataTypeStr=Inherit: Same as input  ParamDataTypeStr=Inherit: Same as input
  cYr : Gain  Gain=nfs.aero.cYr  SaturateOnIntegerOverflow=on  OutDataTypeStr=Inherit: Same as input  ParamDataTypeStr=Inherit: Same as input
  CY : Outport
  wires:
  Sum2/1 -> CY/1
  R/1 -> cYr/1
  P/1 -> cYp/1
  DeltaRudder/1 -> cYdelta_r/1
  DeltaAileron/1 -> cYdelta_a/1
  Velocity Magnitude/1(Velocity Magnitude) -> 2/1
  Linear Velocity/1 -> Velocity Magnitude/1(Velocity)
  Beta/1 -> cYbeta/1
  CY*b/(2V)/1 -> Sum2/4
  cYdelta_r/1 -> Sum2/3
  cYdelta_a/1 -> Sum2/2
  cYbeta/1 -> Sum2/1
  2/1 -> CY*b/(2V)/3
  Wing span/1 -> CY*b/(2V)/2
  Sum/1 -> CY*b/(2V)/1
  cYr/1 -> Sum/2
  cYp/1 -> Sum/1

== system FlightSim/Forces & Moments/Repository/Control Forces/Aerodynamic  Force/Wind2Body TM ==
  Alpha : Inport  PortDimensions=1
  Beta : Inport  Port=2  PortDimensions=1
  ChSign : Gain  Gain=-1  SaturateOnIntegerOverflow=on  OutDataTypeStr=Inherit: Same as input  ParamDataTypeStr=Inherit: Same as input
  ChSign1 : Gain  Gain=-1  SaturateOnIntegerOverflow=on  OutDataTypeStr=Inherit: Same as input  ParamDataTypeStr=Inherit: Same as input
  ChSign2 : Gain  Gain=-1  SaturateOnIntegerOverflow=on  OutDataTypeStr=Inherit: Same as input  ParamDataTypeStr=Inherit: Same as input
  Product{,1..3} (4 alike) : Product  SaturateOnIntegerOverflow=on  InputSameDT=on  OutDataTypeStr=Inherit: Same as first input
  S Matrix : Concatenate  NumInputs=3  Mode=Multidimensional array  ConcatenateDimension=2
  S Col1 : Concatenate  NumInputs=3  Mode=Multidimensional array
  S Col2 : Concatenate  NumInputs=3  Mode=Multidimensional array
  S Col3 : Concatenate  NumInputs=3  Mode=Multidimensional array
  Trigonometric Function : Trigonometry
  Trigonometric Function1 : Trigonometry  Operator=cos
  Trigonometric Function2 : Trigonometry
  Trigonometric Function3 : Trigonometry  Operator=cos
  Zero : Constant  Value=0
  T_BW : Outport  PortDimensions=[3,3]
  wires:
  S Matrix/1 -> T_BW/1
  S Col3/1 -> S Matrix/3
  S Col2/1 -> S Matrix/2
  S Col1/1 -> S Matrix/1
  ChSign2/1 -> S Col3/2
  Product2/1 -> S Col3/1
  Product3/1 -> ChSign2/1
  Zero/1 -> S Col2/3
  ChSign1/1 -> S Col1/3
  ChSign/1 -> S Col1/2
  Product/1 -> S Col1/1
  Product1/1 -> ChSign/1
  Trigonometric Function3/1 -> Product2/2, S Col2/2, Product/2
  Trigonometric Function2/1 -> Product3/2, S Col2/1, Product1/2
  Trigonometric Function1/1 -> Product/1, S Col3/3, Product1/1
  Trigonometric Function/1 -> Product3/1, Product2/1, ChSign1/1
  Beta/1 -> Trigonometric Function2/1, Trigonometric Function3/1
  Alpha/1 -> Trigonometric Function1/1, Trigonometric Function/1

== system FlightSim/Forces & Moments/Repository/Forces/Aerodynamic  Force/Wind2Body TM ==
  Alpha : Inport  PortDimensions=1
  Beta : Inport  Port=2  PortDimensions=1
  ChSign : Gain  Gain=-1  SaturateOnIntegerOverflow=on  OutDataTypeStr=Inherit: Same as input  ParamDataTypeStr=Inherit: Same as input
  ChSign1 : Gain  Gain=-1  SaturateOnIntegerOverflow=on  OutDataTypeStr=Inherit: Same as input  ParamDataTypeStr=Inherit: Same as input
  ChSign2 : Gain  Gain=-1  SaturateOnIntegerOverflow=on  OutDataTypeStr=Inherit: Same as input  ParamDataTypeStr=Inherit: Same as input
  Product{,1..3} (4 alike) : Product  SaturateOnIntegerOverflow=on  InputSameDT=on  OutDataTypeStr=Inherit: Same as first input
  S Matrix : Concatenate  NumInputs=3  Mode=Multidimensional array  ConcatenateDimension=2
  S Col1 : Concatenate  NumInputs=3  Mode=Multidimensional array
  S Col2 : Concatenate  NumInputs=3  Mode=Multidimensional array
  S Col3 : Concatenate  NumInputs=3  Mode=Multidimensional array
  Trigonometric Function : Trigonometry
  Trigonometric Function1 : Trigonometry  Operator=cos
  Trigonometric Function2 : Trigonometry
  Trigonometric Function3 : Trigonometry  Operator=cos
  Zero : Constant  Value=0
  T_BW : Outport  PortDimensions=[3,3]
  wires:
  S Matrix/1 -> T_BW/1
  S Col3/1 -> S Matrix/3
  S Col2/1 -> S Matrix/2
  S Col1/1 -> S Matrix/1
  ChSign2/1 -> S Col3/2
  Product2/1 -> S Col3/1
  Product3/1 -> ChSign2/1
  Zero/1 -> S Col2/3
  ChSign1/1 -> S Col1/3
  ChSign/1 -> S Col1/2
  Product/1 -> S Col1/1
  Product1/1 -> ChSign/1
  Trigonometric Function3/1 -> Product2/2, S Col2/2, Product/2
  Trigonometric Function2/1 -> Product3/2, S Col2/1, Product1/2
  Trigonometric Function1/1 -> Product/1, S Col3/3, Product1/1
  Trigonometric Function/1 -> Product3/1, Product2/1, ChSign1/1
  Beta/1 -> Trigonometric Function2/1, Trigonometric Function3/1
  Alpha/1 -> Trigonometric Function1/1, Trigonometric Function/1

== system FlightSim/Forces & Moments/Repository/Forces/Lift Coefficient/Velocity Magnitude ==
  Velocity : Inport
  Dot Product : DotProduct  InputSameDT=on  OutDataTypeStr=Inherit: Inherit via internal rule
  Sqrt : Sqrt  SaturateOnIntegerOverflow=on
  Velocity Magnitude : Outport
  wires:
  Sqrt/1 -> Velocity Magnitude/1  "abs(V)"
  Velocity/1 -> Dot Product/2, Dot Product/1
  Dot Product/1 -> Sqrt/1

== system FlightSim/Forces & Moments/Repository/Forces/SideForce Coefficient/Velocity Magnitude ==
  Velocity : Inport
  Dot Product : DotProduct  InputSameDT=on  OutDataTypeStr=Inherit: Inherit via internal rule
  Sqrt : Sqrt  SaturateOnIntegerOverflow=on
  Velocity Magnitude : Outport
  wires:
  Sqrt/1 -> Velocity Magnitude/1  "abs(V)"
  Velocity/1 -> Dot Product/2, Dot Product/1
  Dot Product/1 -> Sqrt/1
